simulink model "WPT_18b"  (R2018b)
settings: Solver=VariableStepAuto  StartTime=0.0  StopTime=5  RelTol=1e-3
values from neighbouring files (symbols this model uses):
  C1 = 1/(4*pi*pi*f*f*L1)    [LoadSelfInductance.m]    (also in WPT_SCRIPT_OPTIMAL_Freq.m; WPT_SCRIPT_OPTIMAL_voltage.m = 6.74611055465e-07)
  C2 = 1/(4*pi*pi*f*f*L2)    [LoadSelfInductance.m]    (also in WPT_SCRIPT_OPTIMAL_Freq.m; WPT_SCRIPT_OPTIMAL_voltage.m = 6.74611055465e-07)
  Inverter_period = 1/f    [LoadSelfInductance.m]    (also in WPT_SCRIPT_OPTIMAL_Freq.m; WPT_SCRIPT_OPTIMAL_voltage.m = 0.0001)
  Inverter_phase_delay = Inverter_period/2    [LoadSelfInductance.m]    (also in WPT_SCRIPT_OPTIMAL_Freq.m; WPT_SCRIPT_OPTIMAL_voltage.m = 5e-05)
  L1 = 375.48e-6    (= 0.00037548)    [LoadSelfInductance.m]    (also in WPT_SCRIPT_OPTIMAL_Freq.m; WPT_SCRIPT_OPTIMAL_voltage.m)
  L2 = 375.48e-6    (= 0.00037548)    [LoadSelfInductance.m]    (also in WPT_SCRIPT_OPTIMAL_Freq.m; WPT_SCRIPT_OPTIMAL_voltage.m)
undefined symbols (not defined in the file or in its folder): Ion, Lithium
libraries: powerlib x30, powerlib_meascontrol x4, eePowerMeasurement x2, electricdrivelib x1
settings Model: OrderedModelArguments=off  Creator=DELL  LastModifiedBy=DELL
settings DataIOCC: ReturnWorkspaceOutputs=on

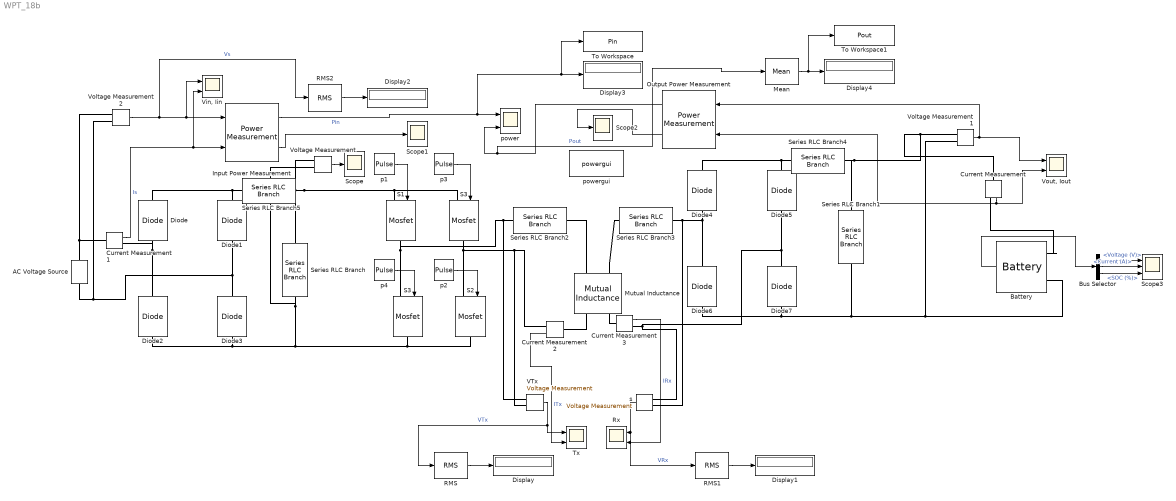
== system WPT_18b ==
  AC Voltage Source : powerlib/Electrical Sources/AC Voltage Source  Amplitude=398  Phase=0  Frequency=60  SampleTime=0  Measurements=None  BusType=swing  Pref=10e3  Qref=0  Qmin=-inf  Qmax=+inf
      settings: SourceProductName=Simscape Electrical
  Battery : electricdrivelib/Extra Sources/Battery  BatType=Lithium-Ion  ShowTempParam=off  ThermalPreset=no  ShowAgeParam=off  NomV=170  NomQ=3  SOC=50  Batt_Tr=30  PresetModel=on  MaxQ=3  MinV=127.5  FullV=197.8778  Dis_rate=1.3043  R=0.56667  Normal_OP=2.713  expZone="[183.6656     0.1473913]"  current=[6.5 13 32.5]  Units=Time  Tci=20  NomT=20  T2=-30  MaxQ2=4.8  FullV2=7.1  Normal_OP2=5.655  expZone2="[6.58           1]"  Rca=0.6  ti=2000  Dp=0  Neq0=0  Tsim=1e6  Ta1=25  Qeol=5.4*0.9  Reol=0.013333*1.2  Char_age=[2.3478, 3]  Dis_age=[2.3478, 10]  N1=1500  N2=10500  N3=1000  N4=1400  Ta2=45  N5=950
      settings: SourceProductName=Simscape Electrical
  Bus Selector : BusSelector  OutputSignals=Voltage (V),Current (A),SOC (%)
  Current Measurement{,1..3} (4 alike) : powerlib/Measurements/Current Measurement  PhasorSimulation=off  OutputType=Complex  PSBequivalent=0
      settings: SourceProductName=Simscape Electrical
  Diode{,1..7} (8 alike) : powerlib/Power Electronics/Diode  Ron=0.001  Lon=0  Vf=0.8  IC=0  UseSnubber=0  Rs=500  Cs=250e-9  Measurements=off
      settings: SourceProductName=Simscape Electrical
  Display{,1..4} (5 alike) : Display
  Input Power Measurement : eePowerMeasurement/Power Measurement  LabelModeActiveChoice=Continuous  F=60  K=[0 1 2 3]  Ts=0
      settings: SourceProductName=Simscape Electrical  SourceProductBaseCode=PS
  Mean : powerlib_meascontrol/Measurements/Mean  Freq=60  Vinit=0  Ts=0
      settings: SourceProductName=Simscape Electrical
  Mutual Inductance : powerlib/Elements/Mutual Inductance  LConnTagsString=a|b  RConnTagsString=A|B  TypeOfMutual=Two or three windings with equal mutual terms  NumberOfWindings=3  SelfImpedance1=[1.1 L1]  SelfImpedance2=[ 1.1 L2]  ThreeWindings=off  SelfImpedance3=[ 1.1 1.1e-03]  MutualImpedance=[1.0 344.58e-06]  InductanceMatrix="[1.0 0.9  0.9 ;  0.9 1.0  0.9;  0.9 0.9 1.0 ] * 1e-3"  ResistanceMatrix="[1.0 0.9  0.9 ;  0.9 1.0  0.9;  0.9 0.9 1.0 ]"  Measurements=None
      settings: AttributesFormatString=\n  SourceProductName=Simscape Electrical  SourceProductBaseCode=PS
  Output Power Measurement : eePowerMeasurement/Power Measurement  LabelModeActiveChoice=Continuous  F=60  K=[0 1 2 3]  Ts=0
      settings: SourceProductName=Simscape Electrical  SourceProductBaseCode=PS
  RMS : powerlib_meascontrol/Measurements/RMS  TrueRMS=on  Freq=5000  RMSInit=0  Ts=0
      settings: SourceProductName=Simscape Electrical
  RMS1 : powerlib_meascontrol/Measurements/RMS  TrueRMS=on  Freq=5000  RMSInit=120  Ts=0
      settings: SourceProductName=Simscape Electrical
  RMS2 : powerlib_meascontrol/Measurements/RMS  TrueRMS=on  Freq=60  RMSInit=120  Ts=0
      settings: SourceProductName=Simscape Electrical
  Rx : Scope  NumInputPorts=2
  S1 : powerlib/Power Electronics/Mosfet  Ron=0.1  Lon=0  Rd=0.01  Vfd=0  IC=0  Rs=1e5  Cs=inf  Measurements=off
      settings: SourceProductName=Simscape Electrical
  S2 : powerlib/Power Electronics/Mosfet  Ron=0.1  Lon=0  Rd=0.01  Vfd=0  IC=0  Rs=1e5  Cs=inf  Measurements=off
      settings: SourceProductName=Simscape Electrical
  S3 : powerlib/Power Electronics/Mosfet  Ron=0.1  Lon=0  Rd=0.01  Vfd=0  IC=0  Rs=1e5  Cs=inf  Measurements=off
      settings: SourceProductName=Simscape Electrical
  "S3 " : powerlib/Power Electronics/Mosfet  Ron=0.1  Lon=0  Rd=0.01  Vfd=0  IC=0  Rs=1e5  Cs=inf  Measurements=off
      settings: SourceProductName=Simscape Electrical
  Scope : Scope
  Scope1 : Scope
  Scope2 : Scope
  Scope3 : Scope  NumInputPorts=3
  Series RLC Branch : powerlib/Elements/Series RLC Branch  LConnTagsString=__new0  RConnTagsString=__new0  BranchType=C  Resistance=1  Inductance=1e-3  SetiL0=off  InitialCurrent=0  Capacitance=3000e-6  Setx0=off  InitialVoltage=0  Measurements=None
      settings: SourceProductName=Simscape Electrical
  Series RLC Branch1 : powerlib/Elements/Series RLC Branch  LConnTagsString=__new0  RConnTagsString=__new0  BranchType=C  Resistance=1  Inductance=1e-3  SetiL0=off  InitialCurrent=0  Capacitance=2000e-6  Setx0=off  InitialVoltage=0  Measurements=None
      settings: SourceProductName=Simscape Electrical
  Series RLC Branch2 : powerlib/Elements/Series RLC Branch  LConnTagsString=__new0  RConnTagsString=__new0  BranchType=C  Resistance=1  Inductance=1e-3  SetiL0=off  InitialCurrent=0  Capacitance=C1  Setx0=on  InitialVoltage=0  Measurements=None
      settings: SourceProductName=Simscape Electrical
  Series RLC Branch3 : powerlib/Elements/Series RLC Branch  LConnTagsString=__new0  RConnTagsString=__new0  BranchType=C  Resistance=1  Inductance=1e-3  SetiL0=off  InitialCurrent=0  Capacitance=C2  Setx0=on  InitialVoltage=0  Measurements=None
      settings: SourceProductName=Simscape Electrical
  Series RLC Branch4 : powerlib/Elements/Series RLC Branch  LConnTagsString=__new0  RConnTagsString=__new0  BranchType=L  Resistance=1  Inductance=300e-3  SetiL0=off  InitialCurrent=0  Capacitance=1e-6  Setx0=off  InitialVoltage=0  Measurements=None
      settings: SourceProductName=Simscape Electrical
  Series RLC Branch5 : powerlib/Elements/Series RLC Branch  LConnTagsString=__new0  RConnTagsString=__new0  BranchType=L  Resistance=1  Inductance=300e-3  SetiL0=off  InitialCurrent=0  Capacitance=1e-6  Setx0=off  InitialVoltage=0  Measurements=None
      settings: SourceProductName=Simscape Electrical
  To Workspace : ToWorkspace  VariableName=Pin  SaveFormat=Timeseries  SampleTime=-1
  To Workspace1 : ToWorkspace  VariableName=Pout  SaveFormat=Timeseries  SampleTime=-1
  Tx : Scope  NumInputPorts=2
  VTx : powerlib/Measurements/Voltage Measurement  PhasorSimulation=off  OutputType=Complex  PSBequivalent=0
      settings: SourceProductName=Simscape Electrical
  "Vin, Iin" : Scope  NumInputPorts=2
  Voltage Measurement : powerlib/Measurements/Voltage Measurement  PhasorSimulation=off  OutputType=Complex  PSBequivalent=0
      settings: SourceProductName=Simscape Electrical
  Voltage Measurement1 : powerlib/Measurements/Voltage Measurement  PhasorSimulation=off  OutputType=Complex  PSBequivalent=0
      settings: SourceProductName=Simscape Electrical
  Voltage Measurement2 : powerlib/Measurements/Voltage Measurement  PhasorSimulation=off  OutputType=Complex  PSBequivalent=0
      settings: SourceProductName=Simscape Electrical
  "Vout, Iout" : Scope  NumInputPorts=2
  p1 : DiscretePulseGenerator  PulseType=Time based  Period=Inverter_period  PulseWidth=50
  p2 : DiscretePulseGenerator  PulseType=Time based  Period=Inverter_period  PulseWidth=50
  p3 : DiscretePulseGenerator  PulseType=Time based  Period=Inverter_period  PulseWidth=50  PhaseDelay=Inverter_phase_delay
  p4 : DiscretePulseGenerator  PulseType=Time based  Period=Inverter_period  PulseWidth=50  PhaseDelay=Inverter_phase_delay
  power : Scope  NumInputPorts=2
  powergui : powerlib/powergui  Priority=1  SimulationMode=Continuous  SampleTime=50e-6  frequency=60  Iterations=50  frequencyindice=60  Pbase=100e6  ErrMax=1e-4  UnitsV=kV  UnitsW=MW  buscounter=0  FunctionMessages=off  echomessages=off  EnableUseOfTLC=off  CurrentSourceSwitches=off  DisableSnubberDevices=off  DisableRonSwitches=off  DisableVfSwitches=off  DisplayEquations=off  AutomaticDiscreteSolvers=off  SolverType=Tustin/Backward Euler (TBE)  Interpol=off  ExternalGateDelay=off  methode=off  Ts=100  x0status=blocks  SPID=on  SwTol=0  HookPort=off  NonlinearTolerance=1e-4  nMaxIteration=100  ContinueOnMaxIteration=off  RestoreLinks=warning  ResistiveCurrentMeasurement=off  Frange=[0:2:500]  Ylog=off  Xlog=on  ShowGrid=off  save=off  variable=ZData  structure=0  ZoomFFT=off  StartTime=0.0  cycles=1  DisplayStyle=1  fundamental=60  FreqAxis=off  MaxFrequency=1000  frequencyindicesteady=1  RmsSteady=1  display=off
      settings: SourceProductName=Simscape Electrical
  s : powerlib/Measurements/Voltage Measurement  PhasorSimulation=off  OutputType=Complex  PSBequivalent=0
      settings: SourceProductName=Simscape Electrical
  wires:
  p4/1 -> "S3 "/1
  Output Power Measurement/1 -> Mean/1, power/2  "Pout"
  s/1 -> RMS1/1, Rx/1  "VRx"
  Battery/1 -> Bus Selector/1
  Input Power Measurement/1 -> To Workspace/1, Display3/1, power/1  "Pin"
  Current Measurement/1 -> "Vout, Iout"/2, Output Power Measurement/2
  Voltage Measurement2/1 -> RMS2/1, Input Power Measurement/1, "Vin, Iin"/1  "Vs"
  Bus Selector/3 -> Scope3/3  "<SOC (%)>"
  Current Measurement2/1 -> Tx/2  "ITx"
  Current Measurement3/1 -> Rx/2  "IRx"
  p3/1 -> S3/1
  Current Measurement1/1 -> "Vin, Iin"/2, Input Power Measurement/2  "Is"
  p2/1 -> S2/1
  p1/1 -> S1/1
  VTx/1 -> RMS/1, Tx/1  "VTx"
  Voltage Measurement1/1 -> "Vout, Iout"/1, Output Power Measurement/1
  Voltage Measurement/1 -> Scope/1
  Bus Selector/1 -> Scope3/1  "<Voltage (V)>"
  Bus Selector/2 -> Scope3/2  "<Current (A)>"
  RMS/1 -> Display/1
  RMS1/1 -> Display1/1
  RMS2/1 -> Display2/1
  Mean/1 -> To Workspace1/1, Display4/1
  Input Power Measurement/2 -> Scope1/1
  Output Power Measurement/2 -> Scope2/1
  connections:
  S3/LConn1 -- Voltage Measurement/LConn1 -- Series RLC Branch/LConn1 -- Series RLC Branch5/RConn1 -- S1/LConn1
  Voltage Measurement1/LConn1 -- Series RLC Branch1/LConn1 -- Series RLC Branch4/RConn1 -- Current Measurement/LConn1
  Diode5/RConn1 -- Series RLC Branch4/LConn1 -- Diode4/RConn1
  Diode7/RConn1 -- Diode5/LConn1 -- s/LConn2 -- Current Measurement3/RConn1
  VTx/LConn2 -- S2/LConn1 -- S3/RConn1 -- Current Measurement2/RConn1
  Diode2/RConn1 -- Diode/LConn1 -- Current Measurement1/RConn1
  Current Measurement1/LConn1 -- AC Voltage Source/RConn1 -- Voltage Measurement2/LConn1
  Diode3/LConn1 -- Diode2/LConn1 -- S2/RConn1 -- "S3 "/RConn1 -- Series RLC Branch/RConn1 -- Voltage Measurement/LConn2
  AC Voltage Source/LConn1 -- Diode1/LConn1 -- Diode3/RConn1 -- Voltage Measurement2/LConn2
  Diode1/RConn1 -- Diode/RConn1 -- Series RLC Branch5/LConn1
  Series RLC Branch2/LConn1 -- S1/RConn1 -- "S3 "/LConn1 -- VTx/LConn1
  Voltage Measurement1/LConn2 -- Diode7/LConn1 -- Diode6/LConn1 -- Series RLC Branch1/RConn1 -- Battery/LConn2
  Series RLC Branch3/RConn1 -- Diode4/LConn1 -- Diode6/RConn1 -- s/LConn1
  Current Measurement2/LConn1 -- Mutual Inductance/RConn1
  Mutual Inductance/RConn2 -- Current Measurement3/LConn1
  Battery/LConn1 -- Current Measurement/RConn1
  Mutual Inductance/LConn2 -- Series RLC Branch3/LConn1
  Mutual Inductance/LConn1 -- Series RLC Branch2/RConn1
